simulink model "PID"  (R2020a)
settings: Solver=VariableStepAuto  StartTime=0.0  StopTime=10.0  RelTol=1e-3
settings Model: Creator=Ishan's PC  LastModifiedBy=Ishan's PC

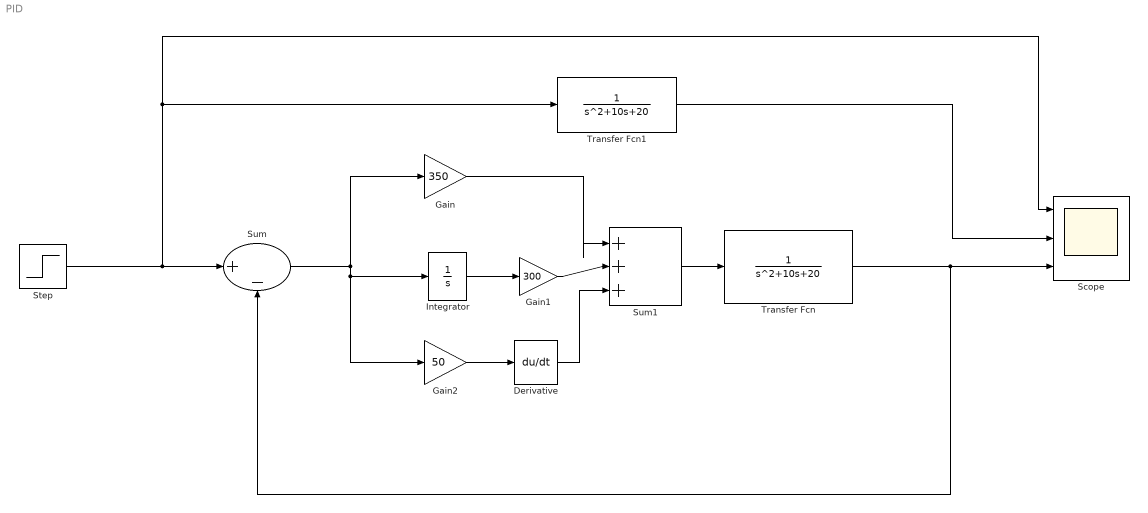
== system PID ==
  Derivative : Derivative
  Gain : Gain  Gain=350
  Gain1 : Gain  Gain=300
  Gain2 : Gain  Gain=50
  Integrator : Integrator
  Scope : Scope  NumInputPorts=3
  Step : Step  SampleTime=0
  Sum : Sum  Inputs=|+-
  Sum1 : Sum  Inputs=|+++
  Transfer Fcn : TransferFcn  Denominator=[1 10 20]
  Transfer Fcn1 : TransferFcn  Denominator=[1 10 20]
  wires:
  Step/1 -> Transfer Fcn1/1, Scope/1, Sum/1
  Transfer Fcn/1 -> Sum/2, Scope/3
  Transfer Fcn1/1 -> Scope/2
  Sum/1 -> Gain2/1, Integrator/1, Gain/1
  Integrator/1 -> Gain1/1
  Gain1/1 -> Sum1/2
  Gain/1 -> Sum1/1
  Gain2/1 -> Derivative/1
  Derivative/1 -> Sum1/3
  Sum1/1 -> Transfer Fcn/1
